simulink model "HEV_ECMS"  (Simulink 10.2)
settings: Solver=FixedStepDiscrete  StartTime=0.0  StopTime=400  FixedStep=data.dt  RelTol=1e-3  EnableMultiTasking=on
InitFcn:
  | init_HEV_ECMS
StopFcn:
  | if t(end)==str2num(get_param(char(bdroot(gcb)),'StopTime'))
  | msgbox('Simulation completed')
  | else
  | msgbox('Simulation aborted due to limitation in one of the components','','error')
  | end
undefined symbols (not defined in the file or in its folder): DiscIntNeverNeededParam, MATLAB_to_Python
undefined symbols (not defined in the file): data
libraries: simulink x7, qss_tb_library x3, pid_lib x1
settings Model: Creator=oberg  LastModifiedBy=ruchitbhikadiya  ExtModeAutoUpdateStatusClock=off
settings DataIOCC: LimitDataPoints=on
settings OptimizationCC: ExpressionDepthLimit=2147483647  InitFltsAndDblsToZero=on
settings DebuggingCC: SaveWithParameterizedLinksMsg=none  SignalResolutionControl=TryResolveAllWithWarning  SolverPrmCheckMsg=warning  MultiTaskDSMMsg=warning  MultiTaskCondExecSysMsg=none  StateNameClashWarn=warning
settings GRTTargetCC: TargetFcnLib=ansi_tfl_tmw.mat
settings ConfigComp: CovSFcnEnable=off

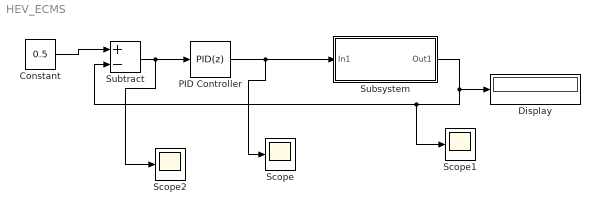
== system HEV_ECMS ==
  Constant : Constant  Value=0.5
  Display : Display
  PID Controller : pid_lib/PID Controller  Controller=PID  Form=Parallel  TimeDomain=Discrete-time  UseExternalTs=off  SampleTime=-1  IntegratorMethod=Forward Euler  FilterMethod=Forward Euler  ControllerParametersSource=internal  P=25  I=0.06  D=0.004  UseFilter=off  N=100  TunerSelectOption=Transfer Function Based (PID Tuner App)  InitialConditionSource=internal  InitialConditionForIntegrator=0  InitialConditionForFilter=0  DifferentiatorICPrevScaledInput=0  ExternalReset=none  TrackingMode=off  Kt=1  LimitOutput=off  SatLimitsSource=internal  UpperSaturationLimit=inf  LowerSaturationLimit=-inf  LinearizeAsGain=on  AntiWindupMode=none  Kb=1  POutMin=[]  POutMax=[]  IOutMin=[]  IOutMax=[]  DOutMin=[]  DOutMax=[]  NOutMin=[]  NOutMax=[]  SumOutMin=[]  SumOutMax=[]  SaturationOutMin=[]  SaturationOutMax=[]  PParamMin=[]  PParamMax=[]  IParamMin=[]  IParamMax=[]  DParamMin=[]  DParamMax=[]  NParamMin=[]  NParamMax=[]  KbParamMin=[]  KbParamMax=[]  KtParamMin=[]  KtParamMax=[]  KbOutMin=[]  KbOutMax=[]  KtOutMin=[]  KtOutMax=[]  IntegratorOutMin=[]  IntegratorOutMax=[]  FilterOutMin=[]  FilterOutMax=[]  SumI1OutMin=[]  SumI1OutMax=[]  SumI2OutMin=[]  SumI2OutMax=[]  SumI3OutMin=[]  SumI3OutMax=[]  SumI4OutMin=[]  SumI4OutMax=[]  SumDOutMin=[]  SumDOutMax=[]  DifferentiatorOutMin=[]  DifferentiatorOutMax=[]  FilterDiffOutCoefMin=[]  FilterDiffOutCoefMax=[]  ReciprocalOutMin=[]  ReciprocalOutMax=[]  SumDenOutMin=[]  SumDenOutMax=[]  SumNumOutMin=[]  SumNumOutMax=[]  DivideOutMin=[]  DivideOutMax=[]  UdiffTsProdOutMin=[]  UdiffTsProdOutMax=[]  NTsProdOutMin=[]  NTsProdOutMax=[]  UintegralTsProdOutMin=[]  UintegralTsProdOutMax=[]  UngainTsProdOutMin=[]  UngainTsProdOutMax=[]  IntegratorContinuousStateAttributes=''  IntegratorStateMustResolveToSignalObject=off  IntegratorRTWStateStorageClass=Auto  FilterContinuousStateAttributes=''  FilterStateMustResolveToSignalObject=off  FilterRTWStateStorageClass=Auto  ParallelPVariant=InternalParameters  IdealPVariant=Disabled  IVariant=InternalParameters  DVariant=InternalParameters  IntegratorVariant=Discrete  SatVariant=Disabled  AWVariant=Passthrough  PCopyVariant=Disabled  TRVariant=Disabled  FdbkBlocksVariant=Forward  IdealPFdbkVariant=Disabled  SatFdbkVariant=Disabled  DerivativeFilterVariant=Differentiator  NVariant=Passthrough  NCopyVariant=Disabled_SignalSpec  FilterICVariant=InternalICsDifferentiator  IntegratorICVariant=InternalICs  ExternalResetVariant=Disabled  TRSumVariant=Passthrough  SumFdbkVariant=Disabled  SumVariant=Sum_PID  TsampFilterVariant=InternalTs  TsampNgainVariant=Passthrough  TsampIntegralVariant=Passthrough  ExternalSaturationOutDataTypeStr=Inherit: Same as second input
  Scope : Scope
  Scope1 : Scope
  Scope2 : Scope
  Subsystem : Subsystem
  Subtract : Sum  Inputs=+-
  wires:
  PID Controller/1 -> Scope/1, Subsystem/1(In1)
  Subsystem/1(Out1) -> Display/1, Scope1/1, Subtract/2
  Constant/1 -> Subtract/1
  Subtract/1 -> Scope2/1, PID Controller/1

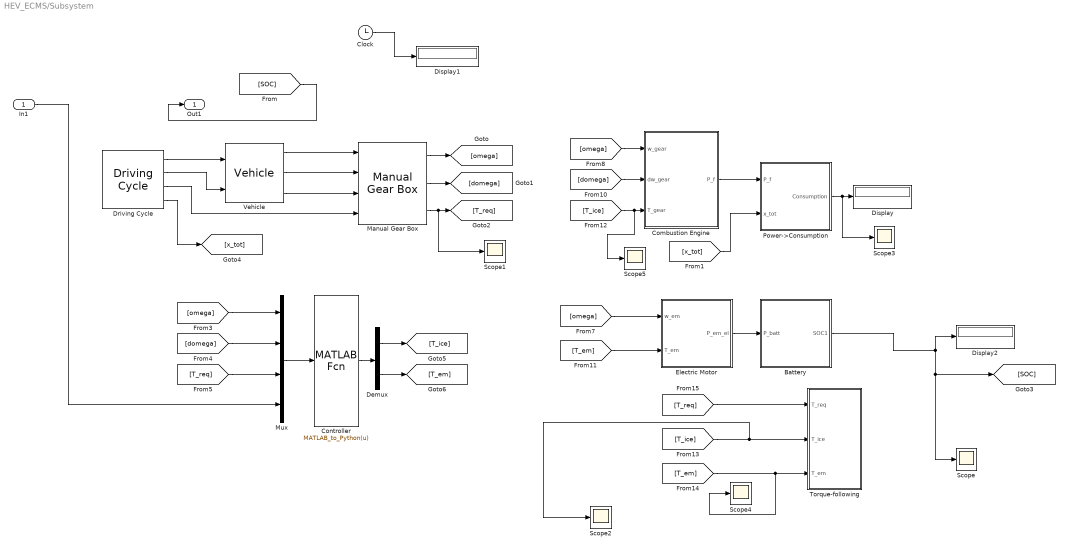
== system HEV_ECMS/Subsystem ==
  In1 : Inport
  Battery : Subsystem  mask{U_oc=data.Uoc, R_i=data.Ri, Q_0=data.Q, SOC_0=0.5, I_max=data.Imax}
      mask prompts: U_oc "Open-Circuit Voltage [V]"; R_i "Inner Resistance [Ohm]"; Q_0 "Capacity [Ah]"; SOC_0 "Initial SOC [-]"; I_max "Max current [I]"
  Clock : Clock
  Combustion Engine : Subsystem
  Controller : MATLABFcn  MATLABFcn=MATLAB_to_Python(u)
  Demux : Demux  Outputs=2
  Display : Display
  Display1 : Display
  Display2 : Display
  Driving Cycle : qss_tb_library/Driving Cycle/Driving Cycle  Tag=cycle  cyclenr=Europe: EUDC manual  stepsize=1  autostop=on
  Electric Motor : Subsystem
  Manual Gear Box : qss_tb_library/Gear System/Manual Gear Box  Tag=transmission  i_1=13.0529  i_2=8.1595  i_3=5.6651  i_4=4.2555  i_5=3.2623  i_diff=1  e_GT=0.98  P_GT0=300  w_wheel_min=1
  Mux : Mux
  Power->Consumption : Subsystem  mask{Hlhv=data.Hlhv, rho_f=data.rho_f}
      mask prompts: Hlhv "Lower Heating Value"; rho_f "Density [kg/m^3]"
  Scope{,1..5} (6 alike) : Scope
  Torque-following : Subsystem
  Vehicle : qss_tb_library/Vehicle/Vehicle  Tag=vehicle  m_f=1500  mt2m_f=0.44  A_f=2.31  r_wheel=0.3  cw=0.32  mu=0.015
  Out1 : Outport
  wires:
  [omega] -> Mux/1
  Demux/2 -> [T_em]
  Manual Gear Box/3 -> Scope1/1, [T_req]
  Vehicle/2 -> Manual Gear Box/2
  Driving Cycle/2 -> Vehicle/2
  Vehicle/3 -> Manual Gear Box/3
  [domega] -> Combustion Engine/2(dw_gear)
  Battery/1(SOC1) -> Scope/1, [SOC], Display2/1
  [x_tot] -> Power->Consumption/2(x_tot)
  Manual Gear Box/1 -> [omega]
  [T_req] -> Torque-following/1(T_req)
  Electric Motor/1(P_em_el) -> Battery/1(P_batt)
  Power->Consumption/1(Consumption) -> Scope3/1, Display/1
  [domega] -> Mux/2
  [T_req] -> Mux/3
  Driving Cycle/1 -> Vehicle/1
  Driving Cycle/3 -> Manual Gear Box/4
  Vehicle/1 -> Manual Gear Box/1
  In1/1 -> Mux/4
  Combustion Engine/1(P_f) -> Power->Consumption/1(P_f)
  Manual Gear Box/2 -> [domega]
  Mux/1 -> Controller/1
  [T_ice] -> Scope5/1, Combustion Engine/3(T_gear)
  Demux/1 -> [T_ice]
  Driving Cycle/4 -> [x_tot]
  [T_ice] -> Scope2/1, Torque-following/2("T_ice ")
  [omega] -> Combustion Engine/1(w_gear)
  [omega] -> Electric Motor/1(w_em)
  [T_em] -> Scope4/1, Torque-following/3(T_em)
  Controller/1 -> Demux/1
  [T_em] -> Electric Motor/2(T_em)
  [SOC] -> Out1/1
  Clock/1 -> Display1/1

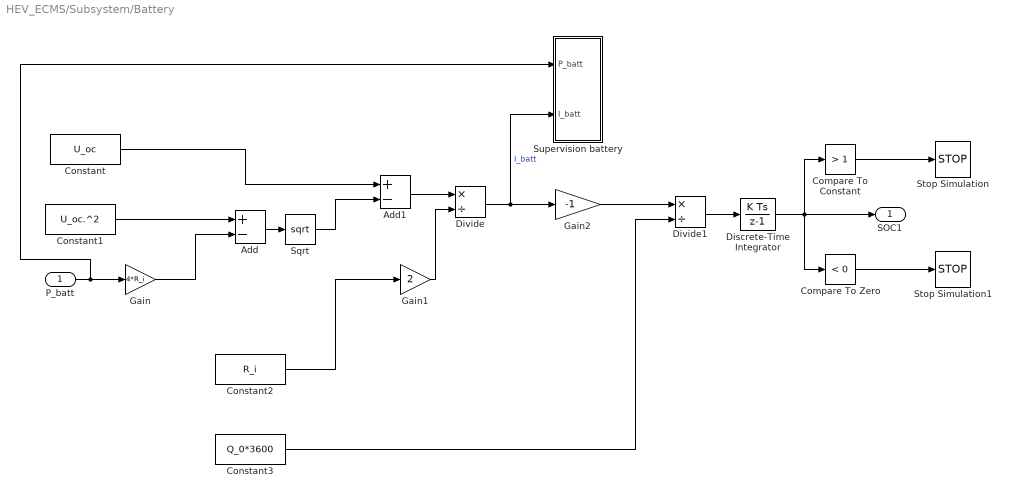
== system HEV_ECMS/Subsystem/Battery ==
  P_batt : Inport
  Add : Sum  Inputs=+-
  Add1 : Sum  Inputs=+-
  Compare To Constant : simulink/Logic and Bit Operations/Compare To Constant  relop=>  const=1  OutDataTypeStr=boolean
  Compare To Zero : simulink/Logic and Bit Operations/Compare To Zero  relop=<  OutDataTypeStr=boolean
  Constant : Constant  Value=U_oc
  Constant1 : Constant  Value=U_oc.^2
  Constant2 : Constant  Value=R_i
  Constant3 : Constant  Value=Q_0*3600
  Discrete-Time Integrator : DiscreteIntegrator  InitialCondition=SOC_0  SampleTime=-1  ICPrevOutput=DiscIntNeverNeededParam  ICPrevScaledInput=DiscIntNeverNeededParam
  Divide : Product  Inputs=*/
  Divide1 : Product  Inputs=*/
  Gain : Gain  Gain=4*R_i
  Gain1 : Gain  Gain=2
  Gain2 : Gain  Gain=-1
  Sqrt : Sqrt  SaturateOnIntegerOverflow=on
  Stop Simulation : Stop
  Stop Simulation1 : Stop
  Supervision battery : Subsystem  AncestorBlock=qss_tb_library/Energy Buffer/Battery/Battery voltage/Supervision battery
  SOC1 : Outport  VectorParamsAs1DForOutWhenUnconnected=off
  wires:
  P_batt/1 -> Gain/1, Supervision battery/1(P_batt)
  Constant1/1 -> Add/1
  Gain/1 -> Add/2
  Add/1 -> Sqrt/1
  Divide/1 -> Supervision battery/2(I_batt), Gain2/1  "I_batt"
  Divide1/1 -> Discrete-Time Integrator/1
  Sqrt/1 -> Add1/2
  Constant/1 -> Add1/1
  Add1/1 -> Divide/1
  Constant2/1 -> Gain1/1
  Gain1/1 -> Divide/2
  Constant3/1 -> Divide1/2
  Gain2/1 -> Divide1/1
  Discrete-Time Integrator/1 -> Compare To Zero/1, SOC1/1, Compare To Constant/1
  Compare To Zero/1 -> Stop Simulation1/1
  Compare To Constant/1 -> Stop Simulation/1

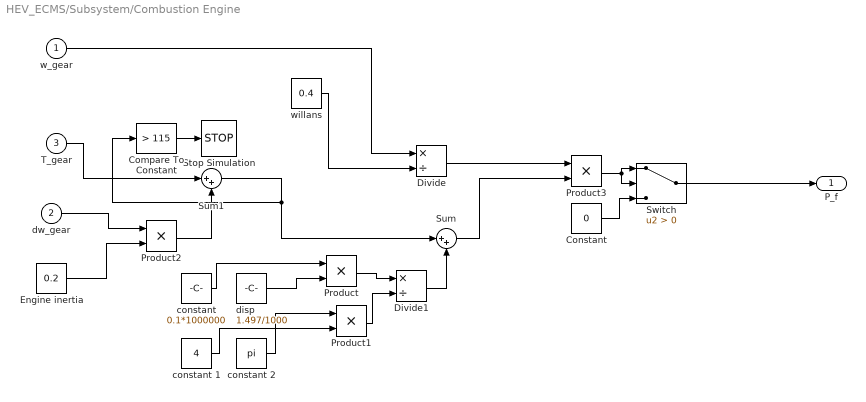
== system HEV_ECMS/Subsystem/Combustion Engine ==
  w_gear : Inport
  dw_gear : Inport  Port=2
  T_gear : Inport  Port=3
  Compare To Constant : simulink/Logic and Bit Operations/Compare To Constant  relop=>  const=115  OutDataTypeStr=boolean
  Constant : Constant  Value=0
  Divide : Product  Inputs=*/
  Divide1 : Product  Inputs=*/
  Engine inertia : Constant  Value=0.2
  Product{,1..3} (4 alike) : Product
  Stop Simulation : Stop
  Sum : Sum  Inputs=|++
  Sum1 : Sum  Inputs=|++
  Switch : Switch  Criteria=u2 > Threshold
  constant : Constant  Value=0.1*1000000
  constant 1 : Constant  Value=4
  constant 2 : Constant  Value=pi
  disp : Constant  Value=1.497/1000
  willans : Constant  Value=0.4
  P_f : Outport  VectorParamsAs1DForOutWhenUnconnected=off
  wires:
  w_gear/1 -> Divide/1
  disp/1 -> Product/2
  constant/1 -> Product/1
  Product/1 -> Divide1/1
  constant 2/1 -> Product1/1
  constant 1/1 -> Product1/2
  Product1/1 -> Divide1/2
  Engine inertia/1 -> Product2/2
  dw_gear/1 -> Product2/1
  Divide/1 -> Product3/1
  willans/1 -> Divide/2
  T_gear/1 -> Sum1/1
  Product2/1 -> Sum1/2
  Sum/1 -> Product3/2
  Sum1/1 -> Compare To Constant/1, Sum/1
  Constant/1 -> Switch/3
  Product3/1 -> Switch/2, Switch/1
  Switch/1 -> P_f/1
  Divide1/1 -> Sum/2
  Compare To Constant/1 -> Stop Simulation/1

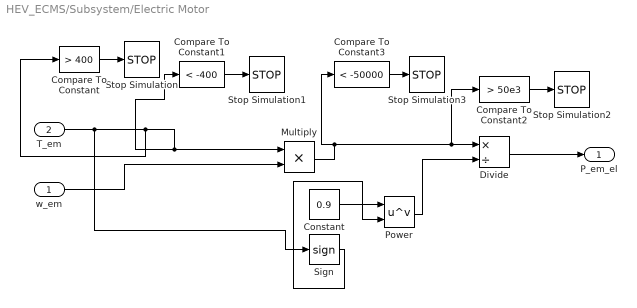
== system HEV_ECMS/Subsystem/Electric Motor ==
  w_em : Inport
  T_em : Inport  Port=2
  Compare To Constant : simulink/Logic and Bit Operations/Compare To Constant  relop=>  const=400  OutDataTypeStr=boolean
  Compare To Constant1 : simulink/Logic and Bit Operations/Compare To Constant  relop=<  const=-400  OutDataTypeStr=boolean
  Compare To Constant2 : simulink/Logic and Bit Operations/Compare To Constant  relop=>  const=50e3  OutDataTypeStr=boolean
  Compare To Constant3 : simulink/Logic and Bit Operations/Compare To Constant  relop=<  const=-50000  OutDataTypeStr=boolean
  Constant : Constant  Value=0.9
  Divide : Product  Inputs=*/
  Multiply : Product
  Power : Math  Operator=pow  SignedPower=on  SaturateOnIntegerOverflow=on
  Sign : Signum
  Stop Simulation{,1..3} (4 alike) : Stop
  P_em_el : Outport  VectorParamsAs1DForOutWhenUnconnected=off
  wires:
  w_em/1 -> Multiply/2
  Constant/1 -> Power/1
  Sign/1 -> Power/2
  Power/1 -> Divide/2
  Divide/1 -> P_em_el/1
  T_em/1 -> Sign/1, Compare To Constant/1, Multiply/1, Compare To Constant1/1
  Multiply/1 -> Compare To Constant2/1, Divide/1, Compare To Constant3/1
  Compare To Constant/1 -> Stop Simulation/1
  Compare To Constant1/1 -> Stop Simulation1/1
  Compare To Constant2/1 -> Stop Simulation2/1
  Compare To Constant3/1 -> Stop Simulation3/1

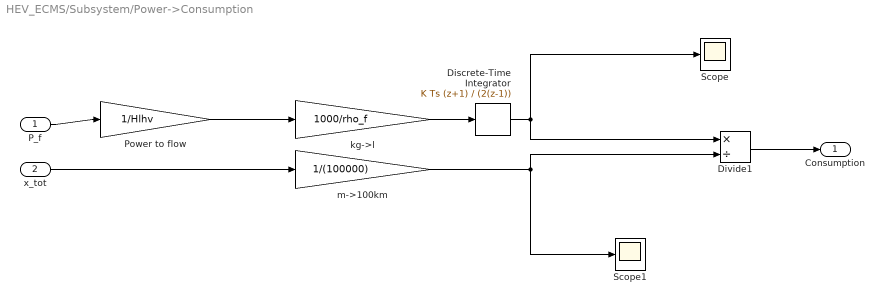
== system HEV_ECMS/Subsystem/Power->Consumption ==
  P_f : Inport
  x_tot : Inport  Port=2
  Discrete-Time Integrator : DiscreteIntegrator  IntegratorMethod=Integration: Trapezoidal  SampleTime=-1  ICPrevOutput=DiscIntNeverNeededParam  ICPrevScaledInput=DiscIntNeverNeededParam
  Divide1 : Product  Inputs=*/
  Power to flow : Gain  Gain=1/Hlhv
  Scope : Scope
  Scope1 : Scope
  kg->l : Gain  Gain=1000/rho_f
  m->100km : Gain  Gain=1/(100000)
  Consumption : Outport  VectorParamsAs1DForOutWhenUnconnected=off
  wires:
  Divide1/1 -> Consumption/1
  P_f/1 -> Power to flow/1
  Power to flow/1 -> kg->l/1
  kg->l/1 -> Discrete-Time Integrator/1
  x_tot/1 -> m->100km/1
  m->100km/1 -> Divide1/2, Scope1/1
  Discrete-Time Integrator/1 -> Divide1/1, Scope/1

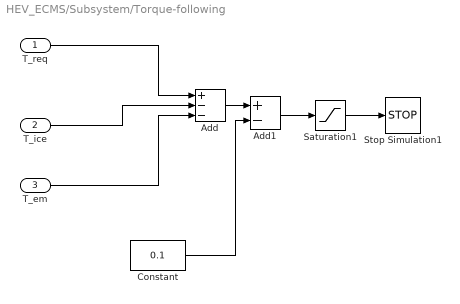
== system HEV_ECMS/Subsystem/Torque-following ==
  T_req : Inport
  "T_ice " : Inport  Port=2
  T_em : Inport  Port=3
  Add : Sum  Inputs=+--
  Add1 : Sum  Inputs=+-
  Constant : Constant  Value=0.1
  Saturation1 : Saturate  UpperLimit=inf  LowerLimit=0
  Stop Simulation1 : Stop
  wires:
  "T_ice "/1 -> Add/2
  T_em/1 -> Add/3
  T_req/1 -> Add/1
  Saturation1/1 -> Stop Simulation1/1
  Add/1 -> Add1/1
  Constant/1 -> Add1/2
  Add1/1 -> Saturation1/1

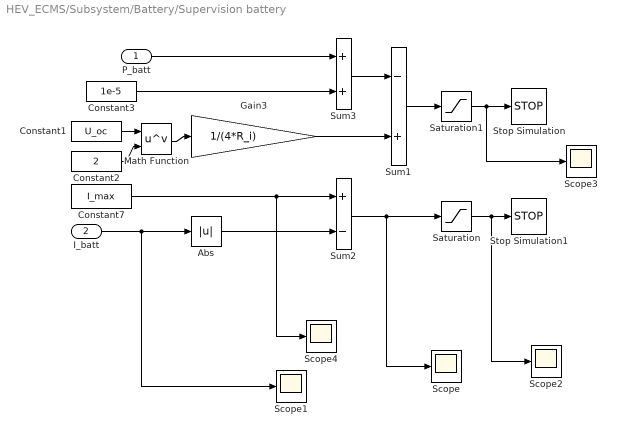
== system HEV_ECMS/Subsystem/Battery/Supervision battery ==
  P_batt : Inport
  I_batt : Inport  Port=2
  Abs : Abs  SaturateOnIntegerOverflow=on
  Constant1 : Constant  Value=U_oc
  Constant2 : Constant  Value=2
  Constant3 : Constant  Value=1e-5
  Constant7 : Constant  Value=I_max
  Gain3 : Gain  Gain=1/(4*R_i)  SaturateOnIntegerOverflow=on  OutDataTypeStr=Inherit: Same as input  ParamDataTypeStr=Inherit: Same as input
  Math Function : Math  Operator=pow  SignedPower=on  SaturateOnIntegerOverflow=on
  Saturation : Saturate  UpperLimit=0  LowerLimit=-inf
  Saturation1 : Saturate  UpperLimit=0  LowerLimit=-inf
  Scope{,1..4} (5 alike) : Scope
  Stop Simulation : Stop
  Stop Simulation1 : Stop
  Sum1 : Sum  Inputs=-+  InputSameDT=on  SaturateOnIntegerOverflow=on  OutDataTypeStr=Inherit: Same as first input
  Sum2 : Sum  Inputs=+-  InputSameDT=on  SaturateOnIntegerOverflow=on  OutDataTypeStr=Inherit: Same as first input
  Sum3 : Sum  InputSameDT=on  SaturateOnIntegerOverflow=on  OutDataTypeStr=Inherit: Same as first input
  wires:
  Abs/1 -> Sum2/2
  I_batt/1 -> Abs/1, Scope1/1
  Sum2/1 -> Saturation/1, Scope/1
  Constant7/1 -> Sum2/1, Scope4/1
  P_batt/1 -> Sum3/1
  Sum1/1 -> Saturation1/1
  Saturation1/1 -> Stop Simulation/1, Scope3/1
  Saturation/1 -> Stop Simulation1/1, Scope2/1
  Gain3/1 -> Sum1/2
  Sum3/1 -> Sum1/1
  Constant1/1 -> Math Function/1
  Math Function/1 -> Gain3/1
  Constant2/1 -> Math Function/2
  Constant3/1 -> Sum3/2
